simulink model "ExtremumSeekingControlExample"  (R2021a)
settings: Solver=FixedStepAuto  StartTime=0.0  StopTime=T  FixedStep=Ts  RelTol=1e-3
values from neighbouring files (symbols this model uses):
  Ki = 0.0025    [ExtremumSeekingControlExample_m.m]
  Ts = 0.1    [ExtremumSeekingControlExample_m.m]
  w_A = 0.5    [ExtremumSeekingControlExample_m.m]
  x_off = 5    [ExtremumSeekingControlExample_m.m]
  y_off = -10    [ExtremumSeekingControlExample_m.m]
libraries: DRC_SimulinkLibrary x1
settings Model: Creator=sebastiaanmuld  LastModifiedBy=Sebastiaan
settings SolverCC: AlgebraicLoopSolver=TrustRegion

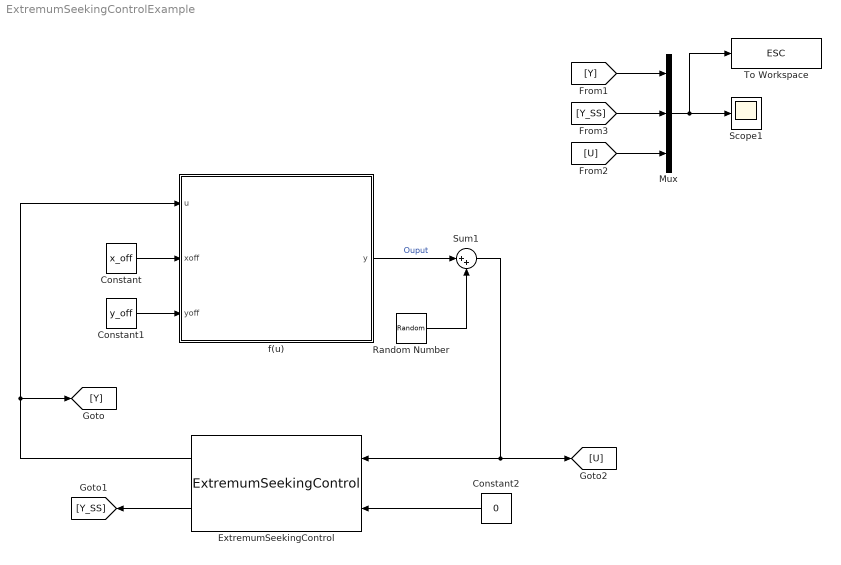
== system ExtremumSeekingControlExample ==
  Constant : Constant  Value=x_off
  Constant1 : Constant  Value=y_off
  Constant2 : Constant  Value=0
  ExtremumSeekingControl : DRC_SimulinkLibrary/ExtremumSeekingControl  D_A=D_w  D_w=D_A  M_phi=M_phi  Ki=Ki  LPF_wc=F.wcLPF  HPF_wc=F.wcHPF  Ts=Ts
  Mux : Mux  Inputs=3
  Random Number : RandomNumber  Variance=w_A  SampleTime=Ts
  Scope1 : Scope
  Sum1 : Sum  Inputs=|++
  To Workspace : ToWorkspace  VariableName=ESC  SaveFormat=Timeseries  SampleTime=-1
  f(u) : MATLAB Function  TreatAsAtomicUnit=on
  wires:
  Constant/1 -> f(u)/2(xoff)
  Constant1/1 -> f(u)/3(yoff)
  Random Number/1 -> Sum1/2
  f(u)/1(y) -> Sum1/1  "Ouput"
  Sum1/1 -> [U], ExtremumSeekingControl/1
  ExtremumSeekingControl/1 -> [Y], f(u)/1(u)
  Mux/1 -> To Workspace/1, Scope1/1
  [Y] -> Mux/1
  [Y_SS] -> Mux/2
  [U] -> Mux/3
  ExtremumSeekingControl/2 -> [Y_SS]
  Constant2/1 -> ExtremumSeekingControl/2

== matlab function ExtremumSeekingControlExample/f(u) ==
  data: u input; y output; xoff input; yoff input
function y = P(u, xoff, yoff)

    y = -(u-xoff)^2 + yoff;
    
end
